simulink model "f28379D"  (R2023b)
settings: Solver=FixedStepAuto  StartTime=0.0  StopTime=Inf  RelTol=1e-3  EnableMultiTasking=on
values from neighbouring files (symbols this model uses):
  anpha = Vmax^3/(2*Ve*Vmax^2-2*Ve^3)    [dacn_delay.m]
  b1 = 2-(wh*Ts1)^2    (= 1.99975325989)    [dacn_delay.m]
  b2 = -1    [dacn_delay.m]
  b3 = kprv1    [dacn_delay.m]
  b4 = kirv1*Ts1+kprv1*((wh*Ts1)^2-2)    [dacn_delay.m]
  b5 = kprv1-kirv1*Ts1    [dacn_delay.m]
  C = Cmin    [dacn_delay.m]
  c1 = 1    [dacn_delay.m]
  c2 = kpi+kii*Ts/2    [dacn_delay.m]
  c3 = kii*Ts/2-kpi    [dacn_delay.m]
  ki2 = Ve/(sqrt(2)*Pe2)    [dacn_delay.m]
  kv = Vmax/sqrt(2)    [dacn_delay.m]
  m4 = (4*m1/Ts^2+2*m2/Ts+m3)/(4*n1/Ts^2+2*n2/Ts+n3)    [dacn_delay.m]
  m5 = (-8*m1/Ts^2+2*m3)/(4*n1/Ts^2+2*n2/Ts+n3)    [dacn_delay.m]
  m6 = (4*m1/Ts^2-2*m2/Ts+m3)/(4*n1/Ts^2+2*n2/Ts+n3)    [dacn_delay.m]
  n5 = -(-8*n1/Ts^2+2*n3)/(4*n1/Ts^2+2*n2/Ts+n3)    [dacn_delay.m]
  n6 = -(4*n1/Ts^2-2*n2/Ts+n3)/(4*n1/Ts^2+2*n2/Ts+n3)    [dacn_delay.m]
  o = 2*anpha    [dacn_delay.m]
  Ts = 1/20000    (= 5e-05)    [dacn_delay.m]
  Udc = 100    [dacn_delay.m]
  wnom = 2*pi*50    (= 314.159265359)    [dacn_delay.m]
undefined symbols (not defined in the file or in its folder): den_nz1, den_nz2, Down, GPTRIP1SEL, num_nz1, num_nz2, TZ1, Up
libraries: c2802xlib x18, simulink x3, c2837xDlib x2, simulink_extras x1, svdschedulerlib x1, dspsrcs4 x1
(part 2 of 2)

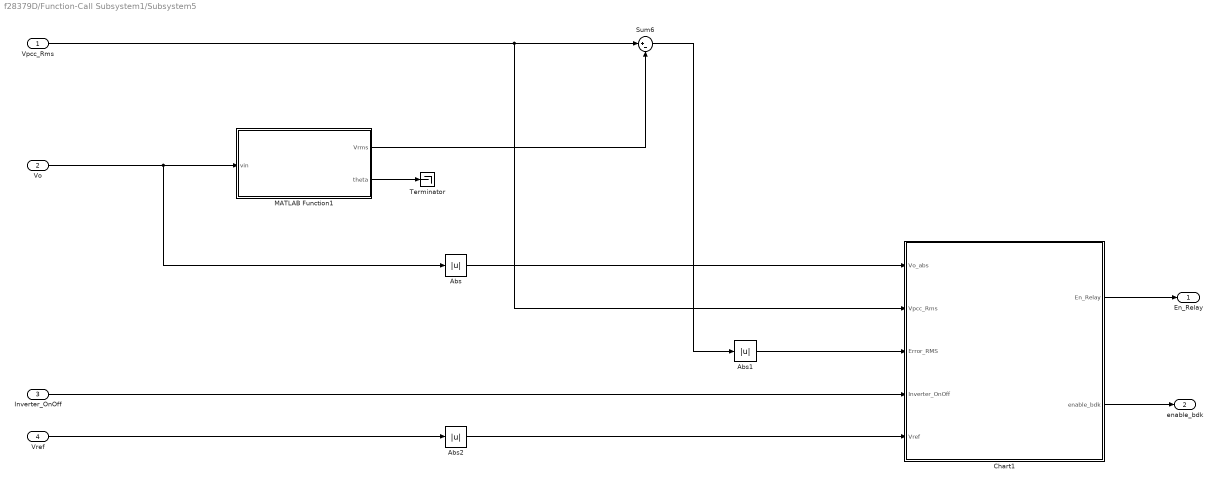
== system f28379D/Function-Call Subsystem1/Subsystem5 ==
  Vpcc_Rms : Inport
  Vo : Inport  Port=2
  Inverter_OnOff : Inport  Port=3
  Vref : Inport  Port=4
  Abs : Abs  SaturateOnIntegerOverflow=off
  Abs1 : Abs  SaturateOnIntegerOverflow=off
  Abs2 : Abs  SaturateOnIntegerOverflow=off
  Chart1 : Stateflow chart  TreatAsAtomicUnit=on
      settings: PortSchema="{\"entries\":[{\"content\":{\"sides\":[{\"content\":{\"connectorIds\":[\"In4\",\"In3\",\"In1\",\"In2\",\"In5\"]},\"type\":\"ConnectorPlacement.EquallySpacedRectSide\",\"uuid\":\"a41d96ef-4339-445d-adf1-46a375c1ebfc\"},{\"content\":{\"connectorIds\":[\"Out1\",\"Out2\"],\"side\":\"RIGHT\"},\"type\":\"ConnectorPlacement.EquallySpacedRectSide\",\"uuid\":\"433b8e1f-da11-4860-b5b3-686501ffdddb\"},{\"content\":{\"side\":\"TOP\"},\"type\":\"ConnectorPlacement.EquallySpacedRectSide\",\"uuid\":\"a76241af-ec7f-4a92-ba0a-9793b7afdcf0\"}]},\"type\":\"ConnectorPlacement.EquallySpacedConnector\",\"uuid\":\"1de099f0-7c57-4924-8764-8a627297889a\"}],\"packageUris\":[\"http://schema.mathworks.com/mf0/Connector/R2020b\"],\"version\":\"1.0\"}"
  MATLAB Function1 : MATLAB Function  TreatAsAtomicUnit=on
  Sum6 : Sum  Inputs=|+-
  Terminator : Terminator
  En_Relay : Outport
  enable_bdk : Outport  Port=2
  wires:
  Vpcc_Rms/1 -> Chart1/3(Vpcc_Rms), Sum6/1
  MATLAB Function1/2(theta) -> Terminator/1
  MATLAB Function1/1(Vrms) -> Sum6/2
  Abs1/1 -> Chart1/1(Error_RMS)
  Vo/1 -> MATLAB Function1/1(vin), Abs/1
  Sum6/1 -> Abs1/1
  Abs/1 -> Chart1/4(Vo_abs)
  Inverter_OnOff/1 -> Chart1/2(Inverter_OnOff)
  Chart1/1(En_Relay) -> En_Relay/1
  Chart1/2(enable_bdk) -> enable_bdk/1
  Vref/1 -> Abs2/1
  Abs2/1 -> Chart1/5(Vref)

== system f28379D/Function-Call Subsystem1/Subsystem6 ==
  vin : Inport
  MATLAB Function2 : MATLAB Function  TreatAsAtomicUnit=on
  Terminator1 : Terminator
  Vpcc_Rms : Outport
  wires:
  MATLAB Function2/2(theta) -> Terminator1/1
  MATLAB Function2/1(Vrms) -> Vpcc_Rms/1
  vin/1 -> MATLAB Function2/1(vin)

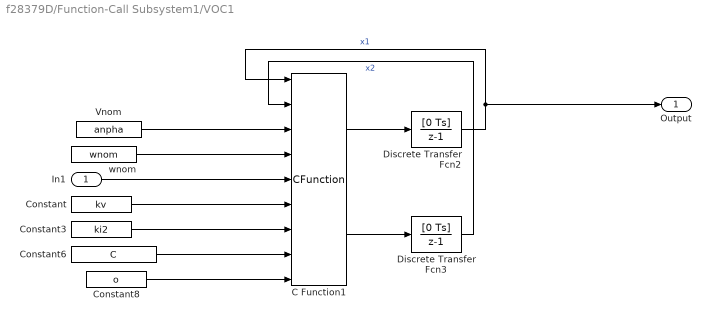
== system f28379D/Function-Call Subsystem1/VOC1 ==
  In1 : Inport
  C Function1 : CFunction  OutputCode=|
      | y1 = (kv*kv*o/anpha-u1*u1-u2*u2)*u1*anpha/(C*kv*kv)-wnom*u2-ki*kv*i/C;
      | y2 = wnom*u1;
  Constant : Constant  Value=kv  OutDataTypeStr=single  SampleTime=-1
  Constant3 : Constant  Value=ki2  OutDataTypeStr=single  SampleTime=-1
  Constant6 : Constant  Value=C  OutDataTypeStr=single  SampleTime=-1
  Constant8 : Constant  Value=o  OutDataTypeStr=single  SampleTime=-1
  Discrete Transfer Fcn2 : DiscreteTransferFcn  Numerator=[0 Ts]  Denominator=[1 -1]  InitialStates=0.5
  Discrete Transfer Fcn3 : DiscreteTransferFcn  Numerator=[0 Ts]  Denominator=[1 -1]  InitialStates=0.5
  Vnom : Constant  Value=anpha  OutDataTypeStr=single  SampleTime=-1
  wnom : Constant  Value=wnom  OutDataTypeStr=single  SampleTime=-1
  Output : Outport
  wires:
  C Function1/1 -> Discrete Transfer Fcn2/1
  Constant/1 -> C Function1/6
  Constant8/1 -> C Function1/9
  C Function1/2 -> Discrete Transfer Fcn3/1
  wnom/1 -> C Function1/4
  Constant3/1 -> C Function1/7
  In1/1 -> C Function1/5
  Discrete Transfer Fcn3/1 -> C Function1/2  "x2"
  Discrete Transfer Fcn2/1 -> C Function1/1, Output/1  "x1"
  Constant6/1 -> C Function1/8
  Vnom/1 -> C Function1/3

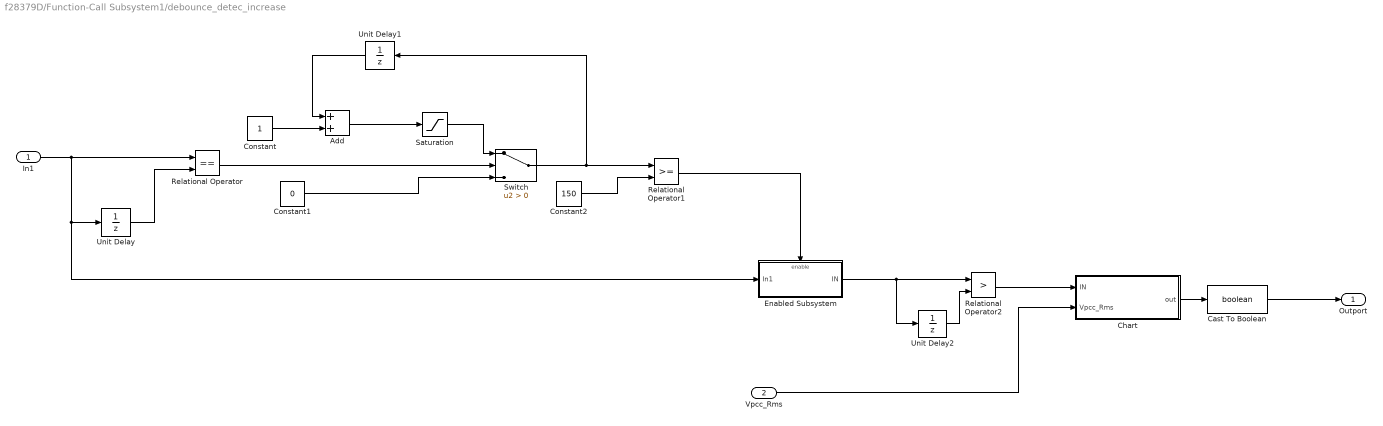
== system f28379D/Function-Call Subsystem1/debounce_detec_increase ==
  In1 : Inport
  Vpcc_Rms : Inport  Port=2
  Add : Sum  OutDataTypeStr=uint8
  Cast To Boolean : DataTypeConversion  OutDataTypeStr=boolean  SaturateOnIntegerOverflow=off  RndMeth=Floor
  Chart : Stateflow chart  TreatAsAtomicUnit=on
  Constant : Constant  OutDataTypeStr=uint8
  Constant1 : Constant  Value=0  OutDataTypeStr=uint8
  Constant2 : Constant  Value=150  OutDataTypeStr=uint8
  Enabled Subsystem : Subsystem  TreatAsAtomicUnit=on
  Relational Operator : RelationalOperator  Operator===  OutDataTypeStr=boolean  RndMeth=Simplest  InputSameDT=off
  Relational Operator1 : RelationalOperator  OutDataTypeStr=boolean  RndMeth=Simplest  InputSameDT=off
  Relational Operator2 : RelationalOperator  Operator=>  OutDataTypeStr=boolean  RndMeth=Simplest  InputSameDT=off
  Saturation : Saturate  UpperLimit=155  LowerLimit=0
  Switch : Switch  Criteria=u2 > Threshold  SaturateOnIntegerOverflow=off  InputSameDT=off
  Unit Delay : UnitDelay  SampleTime=-1  HasFrameUpgradeWarning=on
  Unit Delay1 : UnitDelay  SampleTime=-1  HasFrameUpgradeWarning=on
  Unit Delay2 : UnitDelay  SampleTime=-1  HasFrameUpgradeWarning=on
  Outport : Outport
  wires:
  In1/1 -> Relational Operator/1, Enabled Subsystem/1(In1), Unit Delay/1
  Unit Delay/1 -> Relational Operator/2
  Relational Operator/1 -> Switch/2
  Constant/1 -> Add/2
  Constant1/1 -> Switch/3
  Add/1 -> Saturation/1
  Switch/1 -> Unit Delay1/1, Relational Operator1/1
  Unit Delay1/1 -> Add/1
  Constant2/1 -> Relational Operator1/2
  Relational Operator1/1 -> Enabled Subsystem/Enable
  Enabled Subsystem/1(IN) -> Relational Operator2/1, Unit Delay2/1
  Chart/1(out) -> Cast To Boolean/1
  Saturation/1 -> Switch/1
  Cast To Boolean/1 -> Outport/1
  Unit Delay2/1 -> Relational Operator2/2
  Relational Operator2/1 -> Chart/1(IN)
  Vpcc_Rms/1 -> Chart/2(Vpcc_Rms)

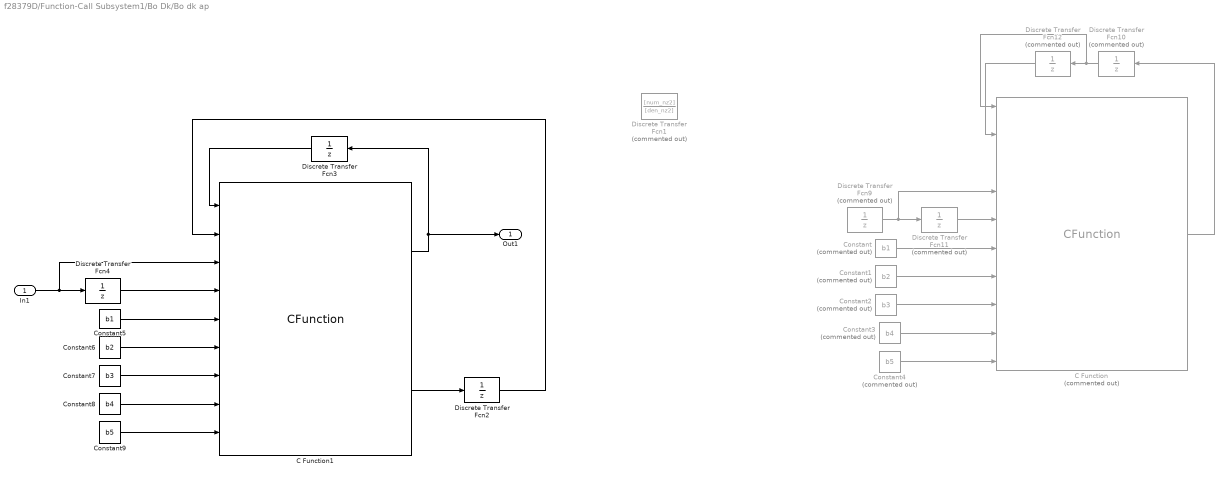
== system f28379D/Function-Call Subsystem1/Bo Dk/Bo dk ap ==
  In1 : Inport  OutDataTypeStr=single
  C Function : CFunction  Commented=on  OutputCode=y_k=b1*y_k_1+b2*y_k_2+b3*u_k+b4*u_k_1+b5*u_k_2;
  C Function1 : CFunction  OutputCode=|
      | y_k=b3*u_k+v_k_1;
      | v_k=b1*y_k+b2*y_k_1+b4*u_k+b5*u_k_1;
  Constant : Constant  Commented=on  Value=b1  OutDataTypeStr=single  SampleTime=-1
  Constant1 : Constant  Commented=on  Value=b2  OutDataTypeStr=single  SampleTime=-1
  Constant2 : Constant  Commented=on  Value=b3  OutDataTypeStr=single  SampleTime=-1
  Constant3 : Constant  Commented=on  Value=b4  OutDataTypeStr=single  SampleTime=-1
  Constant4 : Constant  Commented=on  Value=b5  OutDataTypeStr=single  SampleTime=-1
  Constant5 : Constant  Value=b1  OutDataTypeStr=single  SampleTime=-1
  Constant6 : Constant  Value=b2  OutDataTypeStr=single  SampleTime=-1
  Constant7 : Constant  Value=b3  OutDataTypeStr=single  SampleTime=-1
  Constant8 : Constant  Value=b4  OutDataTypeStr=single  SampleTime=-1
  Constant9 : Constant  Value=b5  OutDataTypeStr=single  SampleTime=-1
  Discrete Transfer Fcn1 : DiscreteTransferFcn  Commented=on  Numerator=[num_nz2]  Denominator=[den_nz2]
  Discrete Transfer Fcn{9..12} (4 alike) : DiscreteTransferFcn  Commented=on  Denominator=[1 0]
  Discrete Transfer Fcn2 : DiscreteTransferFcn  Denominator=[1 0]
  Discrete Transfer Fcn3 : DiscreteTransferFcn  Denominator=[1 0]
  Discrete Transfer Fcn4 : DiscreteTransferFcn  Denominator=[1 0]
  Out1 : Outport  OutDataTypeStr=single
  wires:
  Constant3/1 -> C Function/9
  Constant1/1 -> C Function/7
  Constant4/1 -> C Function/10
  Constant2/1 -> C Function/8
  Discrete Transfer Fcn9/1 -> C Function/4, Discrete Transfer Fcn11/1
  Discrete Transfer Fcn12/1 -> C Function/2
  C Function/1 -> Discrete Transfer Fcn10/1
  Discrete Transfer Fcn10/1 -> Discrete Transfer Fcn12/1, C Function/1
  Discrete Transfer Fcn11/1 -> C Function/5
  Constant/1 -> C Function/6
  C Function1/1 -> Out1/1, Discrete Transfer Fcn3/1
  Discrete Transfer Fcn4/1 -> C Function1/4
  Constant5/1 -> C Function1/5
  Constant6/1 -> C Function1/6
  Constant7/1 -> C Function1/7
  Constant8/1 -> C Function1/8
  Constant9/1 -> C Function1/9
  Discrete Transfer Fcn3/1 -> C Function1/1
  C Function1/2 -> Discrete Transfer Fcn2/1
  Discrete Transfer Fcn2/1 -> C Function1/2
  In1/1 -> C Function1/3, Discrete Transfer Fcn4/1

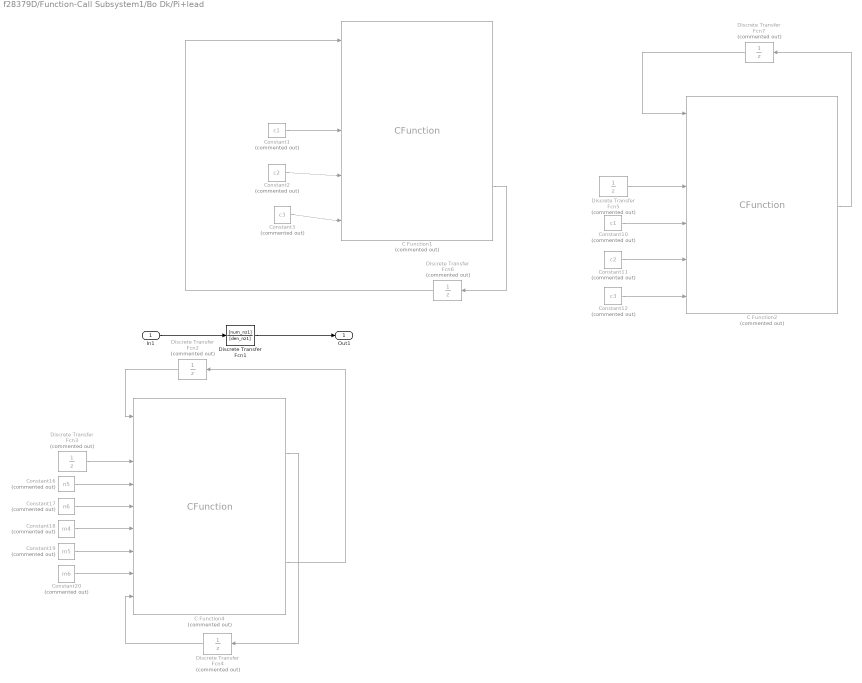
== system f28379D/Function-Call Subsystem1/Bo Dk/Pi+lead ==
  In1 : Inport  OutDataTypeStr=single
  C Function1 : CFunction  Commented=on  OutputCode=|
      | y_k=c2*u_k+v_k_1;
      | v_k=c1*y_k+c3*u_k;
  C Function2 : CFunction  Commented=on  OutputCode=y_k=c1*y_k_1+c2*u_k+c3*u_k_1;
  C Function4 : CFunction  Commented=on  OutputCode=|
      | y_k=m4*u_k+v_k_1;
      | v_k=n5*y_k+n6*y_k_1+m5*u_k+m6*u_k_1;
  Constant1 : Constant  Commented=on  Value=c1  OutDataTypeStr=single  SampleTime=-1
  Constant10 : Constant  Commented=on  Value=c1  OutDataTypeStr=single  SampleTime=-1
  Constant11 : Constant  Commented=on  Value=c2  OutDataTypeStr=single  SampleTime=-1
  Constant12 : Constant  Commented=on  Value=c3  OutDataTypeStr=single  SampleTime=-1
  Constant16 : Constant  Commented=on  Value=n5  OutDataTypeStr=single  SampleTime=-1
  Constant17 : Constant  Commented=on  Value=n6  OutDataTypeStr=single  SampleTime=-1
  Constant18 : Constant  Commented=on  Value=m4  OutDataTypeStr=single  SampleTime=-1
  Constant19 : Constant  Commented=on  Value=m5  OutDataTypeStr=single  SampleTime=-1
  Constant2 : Constant  Commented=on  Value=c2  OutDataTypeStr=single  SampleTime=-1
  Constant20 : Constant  Commented=on  Value=m6  OutDataTypeStr=single  SampleTime=-1
  Constant3 : Constant  Commented=on  Value=c3  OutDataTypeStr=single  SampleTime=-1
  Discrete Transfer Fcn1 : DiscreteTransferFcn  Numerator=[num_nz1]  Denominator=[den_nz1]
  Discrete Transfer Fcn{2..7} (6 alike) : DiscreteTransferFcn  Commented=on  Denominator=[1 0]
  Out1 : Outport  OutDataTypeStr=single
  wires:
  C Function4/1 -> Discrete Transfer Fcn4/1
  C Function4/2 -> Discrete Transfer Fcn2/1
  Discrete Transfer Fcn4/1 -> C Function4/9
  Discrete Transfer Fcn2/1 -> C Function4/1
  Discrete Transfer Fcn3/1 -> C Function4/3
  Constant16/1 -> C Function4/4
  Constant17/1 -> C Function4/5
  Constant18/1 -> C Function4/6
  Constant19/1 -> C Function4/7
  Constant20/1 -> C Function4/8
  Discrete Transfer Fcn7/1 -> C Function2/1
  Constant10/1 -> C Function2/4
  Constant11/1 -> C Function2/5
  Discrete Transfer Fcn5/1 -> C Function2/3
  C Function2/1 -> Discrete Transfer Fcn7/1
  Constant12/1 -> C Function2/6
  Constant1/1 -> C Function1/3
  Constant2/1 -> C Function1/4
  C Function1/2 -> Discrete Transfer Fcn6/1
  Discrete Transfer Fcn6/1 -> C Function1/1
  Constant3/1 -> C Function1/5
  Discrete Transfer Fcn1/1 -> Out1/1
  In1/1 -> Discrete Transfer Fcn1/1

== system f28379D/Function-Call Subsystem1/debounce_detec_increase/Enabled Subsystem ==
  In1 : Inport
  Enable : EnablePort
  IN : Outport
  wires:
  In1/1 -> IN/1

== stateflow chart f28379D/Function-Call Subsystem1/Subsystem5/Chart1 ==
  state OFF
    En_Relay = false;
    enable_bdk = false;
    if (Vpcc_Rms < 10)
    if (Grid_Off < 1000)
    Grid_Off = Grid_Off + 1;
    end
    Grid_On = 0;
    else
    if (Grid_On < 1000)
    Grid_On = Grid_On + 1;
    end
    Grid_Off = 0;
    end
  state On_Normal
    En_Relay = true;
    enable_bdk = true;
  state Pre_Synchronous
    En_Relay = false;
    enable_bdk = true;
    if (Error_RMS < 5)
    if (Change_status < 1000)
    Change_status = Change_status+1;
    end
    else
    Change_status = 0;
    end
  (default) -> OFF
  OFF -> On_Normal [order 1] : [Inverter_OnOff == true && Grid_Off  >= 1000]
      | {Grid_Off =0}
  On_Normal -> OFF : [Inverter_OnOff == false && Vref <1]
  Pre_Synchronous -> On_Normal [order 1] : [Change_status >= 1000 && Vo_abs < 10]
      | {Change_status = 0}
  OFF -> Pre_Synchronous [order 2] : [Inverter_OnOff == true && Grid_On >= 1000]
      | {Grid_On =0}
  Pre_Synchronous -> OFF [order 2] : [Inverter_OnOff == false]
  data: Error_RMS input; Inverter_OnOff input; Vpcc_Rms input; Vo_abs input; En_Relay output =false; Change_status local uint32 =0; Grid_Off local uint32 =0; Grid_On local uint32 =0; enable_bdk output boolean; Vref input

== matlab function f28379D/Function-Call Subsystem1/Subsystem5/MATLAB Function1 ==
  data: vin input; Vrms output; theta output
function [Vrms, theta] = single_phase_rms_phase(vin)
%#codegen

% ép input sang single
vin = single(vin);

% persistent states (single)
persistent v_alpha v_beta
persistent k w Ts

if isempty(v_alpha)
    v_alpha = single(0);
    v_beta  = single(0);

    Ts = single(0.5e-4);          % Sampling time (10 kHz)
    w  = single(2*pi*50);       % 50 Hz
    k  = single(1.414213562);   % sqrt(2)
end

% --- SOGI ---
e = vin - v_alpha;

v_alpha = v_alpha + Ts*( k*w*e - w*v_beta );
v_beta  = v_beta  + Ts*( w*v_alpha );

% --- RMS ---
Vrms = sqrt( (v_alpha*v_alpha + v_beta*v_beta) * single(0.5) );

% --- Phase ---
theta = atan2(v_beta , v_alpha);

% ép output single (an toàn cho codegen)
Vrms  = single(Vrms);
theta = single(theta);

end

== stateflow chart f28379D/Function-Call Subsystem1/debounce_detec_increase/Chart ==
  state OFF
    entry:
    out=0;
  state ON
    out=1;
    if (Vpcc_Rms < 10)
    if (Grid_Off < 10000)
    Grid_Off = Grid_Off + 1;
    end
    else
    Grid_Off = 0;
    end
  (default) -> OFF
  OFF -> ON : [IN==1]
  ON -> OFF : [IN==1 ||...
      | Grid_Off >= 10000]
      | {Grid_Off = 0 }
  data: out output; IN input; Vpcc_Rms input; Grid_Off local uint32 =0

== matlab function f28379D/Function-Call Subsystem1/Subsystem6/MATLAB Function2 ==
  data: vin input; Vrms output; theta output
function [Vrms, theta] = single_phase_rms_phase(vin)
%#codegen

% ép input sang single
vin = single(vin);

% persistent states (single)
persistent v_alpha v_beta
persistent k w Ts

if isempty(v_alpha)
    v_alpha = single(0);
    v_beta  = single(0);

    Ts = single(0.5e-4);          % Sampling time (10 kHz)
    w  = single(2*pi*50);       % 50 Hz
    k  = single(1.414213562);   % sqrt(2)
end

% --- SOGI ---
e = vin - v_alpha;

v_alpha = v_alpha + Ts*( k*w*e - w*v_beta );
v_beta  = v_beta  + Ts*( w*v_alpha );

% --- RMS ---
Vrms = sqrt( (v_alpha*v_alpha + v_beta*v_beta) * single(0.5) );

% --- Phase ---
theta = atan2(v_beta , v_alpha);

% ép output single (an toàn cho codegen)
Vrms  = single(Vrms);
theta = single(theta);

end
